simulink model "AUVModel"  (R2021a)
settings: Solver=FixedStepAuto  StartTime=tStart  StopTime=tStop  FixedStep=tStep  RelTol=1e-3
values from neighbouring files (symbols this model uses):
  dr = 25    [NonlinearProject.m]
  ds = 25    [NonlinearProject.m]
  psiDen = [1, 4.5, 4.4] - psiNum    [NonlinearProject.m]
  psiKd = 0    [NonlinearProject.m]
  psiKi = 0    [NonlinearProject.m]
  psiKp = 1    [NonlinearProject.m]
  psiNum = [0, 1.9, 2.8]    [NonlinearProject.m]
  thetaDen = [1, 4.5, 6, 0.5] - thetaNum    [NonlinearProject.m]
  thetaKd = 0    [NonlinearProject.m]
  thetaKi = 0    [NonlinearProject.m]
  thetaKp = 1    [NonlinearProject.m]
  thetaNum = [0, 0, 1.6, 1.8]    [NonlinearProject.m]
libraries: fod x2
settings Model: Creator=krish  LastModifiedBy=krish

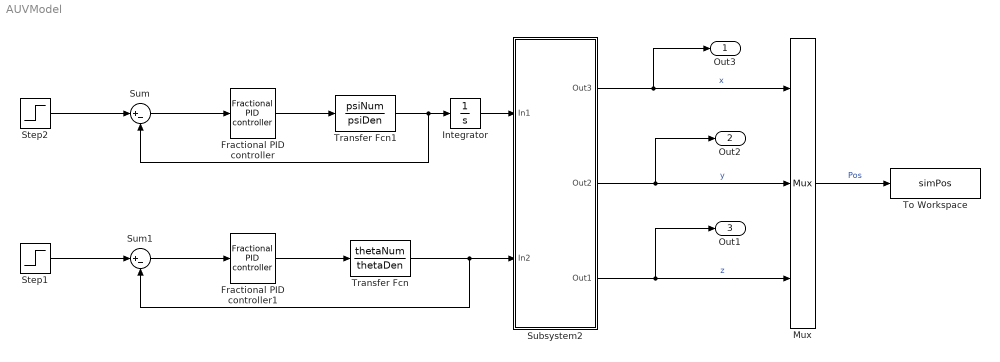
== system AUVModel ==
  Fractional PID controller : fod/Fractional PID controller  Kp=psiKp  Ki=psiKi  lambda=psiLemda  Kd=psiKd  mic=psiMeu  freqRange=[0.001, 1000]  N=5
      settings: SourceProductName=FOMCON Toolbox
  Fractional PID controller1 : fod/Fractional PID controller  Kp=thetaKp  Ki=thetaKi  lambda=thetaLemda  Kd=thetaKd  mic=thetaMeu  freqRange=[0.001, 1000]  N=5
      settings: SourceProductName=FOMCON Toolbox
  Integrator : Integrator
  Mux : Mux  Inputs=3
  Step1 : Step  Time=0  After=(pi/180)*ds  SampleTime=0
  Step2 : Step  Time=0  After=(pi/180)*dr  SampleTime=0
  Subsystem2 : Subsystem
  Sum : Sum  Inputs=|+-
  Sum1 : Sum  Inputs=|+-
  To Workspace : ToWorkspace  VariableName=simPos  SaveFormat=Timeseries  SampleTime=-1
  Transfer Fcn : TransferFcn  Numerator=thetaNum  Denominator=thetaDen
  Transfer Fcn1 : TransferFcn  Numerator=psiNum  Denominator=psiDen
  Out3 : Outport
  Out2 : Outport  Port=2
  Out1 : Outport  Port=3
  wires:
  Integrator/1 -> Subsystem2/1(In1)
  Fractional PID controller/1 -> Transfer Fcn1/1
  Transfer Fcn/1 -> Sum1/2, Subsystem2/2(In2)
  Transfer Fcn1/1 -> Sum/2, Integrator/1
  Fractional PID controller1/1 -> Transfer Fcn/1
  Sum/1 -> Fractional PID controller/1
  Sum1/1 -> Fractional PID controller1/1
  Step2/1 -> Sum/1
  Step1/1 -> Sum1/1
  Subsystem2/1(Out3) -> Mux/1, Out3/1  "x"
  Subsystem2/3(Out1) -> Out1/1, Mux/3  "z"
  Subsystem2/2(Out2) -> Out2/1, Mux/2  "y"
  Mux/1 -> To Workspace/1  "Pos"

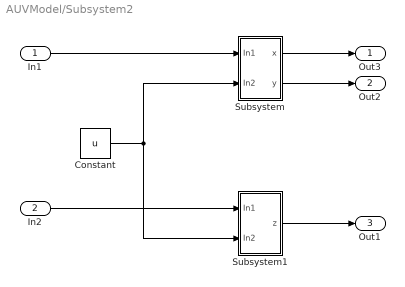
== system AUVModel/Subsystem2 ==
  In1 : Inport
  In2 : Inport  Port=2
  Constant : Constant  Value=u
  Subsystem : Subsystem
  Subsystem1 : Subsystem
  Out3 : Outport
  Out2 : Outport  Port=2
  Out1 : Outport  Port=3
  wires:
  Subsystem/1(x) -> Out3/1
  In2/1 -> Subsystem1/1(In1)
  Constant/1 -> Subsystem/2(In2), Subsystem1/2(In2)
  Subsystem1/1(z) -> Out1/1
  In1/1 -> Subsystem/1(In1)
  Subsystem/2(y) -> Out2/1

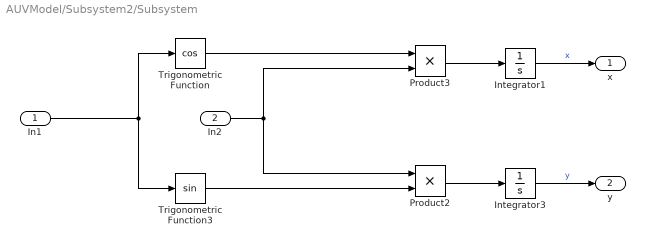
== system AUVModel/Subsystem2/Subsystem ==
  In1 : Inport
  In2 : Inport  Port=2
  Integrator1 : Integrator
  Integrator3 : Integrator
  Product2 : Product
  Product3 : Product
  Trigonometric Function : Trigonometry  Operator=cos
  Trigonometric Function3 : Trigonometry
  x : Outport
  y : Outport  Port=2
  wires:
  In2/1 -> Product3/2, Product2/1
  Integrator1/1 -> x/1  "x"
  Trigonometric Function/1 -> Product3/1
  Product3/1 -> Integrator1/1
  In1/1 -> Trigonometric Function/1, Trigonometric Function3/1
  Integrator3/1 -> y/1  "y"
  Product2/1 -> Integrator3/1
  Trigonometric Function3/1 -> Product2/2

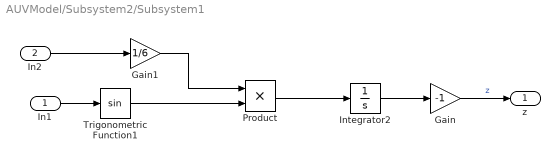
== system AUVModel/Subsystem2/Subsystem1 ==
  In1 : Inport
  In2 : Inport  Port=2
  Gain : Gain  Gain=-1
  Gain1 : Gain  Gain=1/6
  Integrator2 : Integrator
  Product : Product
  Trigonometric Function1 : Trigonometry
  z : Outport
  wires:
  Integrator2/1 -> Gain/1
  In1/1 -> Trigonometric Function1/1
  In2/1 -> Gain1/1
  Product/1 -> Integrator2/1
  Trigonometric Function1/1 -> Product/2
  Gain/1 -> z/1  "z"
  Gain1/1 -> Product/1
